simulink model "Core_Model_Controlled"  (R2023a)
settings: Solver=FixedStepAuto  StartTime=0.0  StopTime=Z  FixedStep=1/24  RelTol=1e-3
values from neighbouring files (symbols this model uses):
  c_eh = 0.85    [Model_Parameters.m]
  C_g = 1    [Model_Parameters.m]
  cc_e = -0.85    [Model_Parameters.m]
  id_a = 0.8*0.028*1.2    (= 0.02688)    [Model_Parameters.m]
  id_g = 0.8*0.072*1.2    (= 0.06912)    [Model_Parameters.m]
  id_l = 0.4*0.139*1.2    (= 0.06672)    [Model_Parameters.m]
  id_r = 0.4*0.428*1.2    (= 0.20544)    [Model_Parameters.m]
  id_z = 0.4*0.33*1.2    (= 0.1584)    [Model_Parameters.m]
  L_a = 0.25    [Model_Parameters.m]
  L_g = 0.1    [Model_Parameters.m]
  L_l = 0.2    [Model_Parameters.m]
  L_r = 0.05    [Model_Parameters.m]
  L_z = 0.08    [Model_Parameters.m]
  R_H2 = 0.05    [Model_Parameters.m]
  R_lh = 0.025    [Model_Parameters.m]
  R_ng = 0.025    [Model_Parameters.m]
  SF_MWh = SF_GWh*1e3    [Main_Script.m]
libraries: fl_lib x120, nesl_utility x93, ee_lib x36, slpidlib x1
(part 3 of 3)

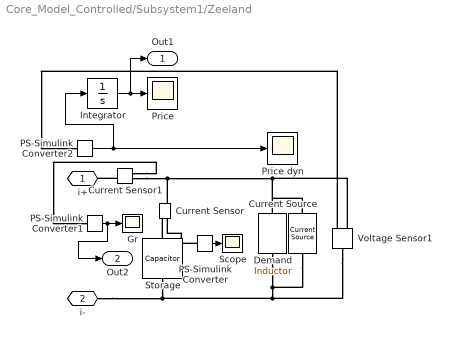
== system Core_Model_Controlled/Subsystem1/Zeeland ==
  Current Sensor : fl_lib/Electrical/Electrical Sensors/Current Sensor
  Current Sensor1 : fl_lib/Electrical/Electrical Sensors/Current Sensor
  Current Source : ee_lib/Sources/Current Source  dc_current=id_z A  ac_current=0 A  ac_shift=0 rad  ac_frequency=0 Hz  noise_mode=ee.enum.sources.noise.Disabled  PSD=0 A^2/Hz  sample_time=1e-3 s  repeatability=ee.enum.sources.repeatability.NotRepeatable  user_seed=0  auto_seed=4168664255  i_specify=off  i_priority=None  i=0 A  i_nominal_specify=off  i_nominal_unit=A  i_nominal_value=1  v_specify=off  v_priority=None  v=0 V  v_nominal_specify=off  v_nominal_unit=V  v_nominal_value=1
  Demand : ee_lib/Passive/Inductor  l=L_z H  enable_L_tol=0  L_tol=20  tol_distribution=1  nSigma=4  r=0 Ohm  g=0 1/Ohm  enable_operating_limits=0  operating_limit_action=2  max_working_current=1 A  power_rating=1 W  enable_faults=ee.enum.enable.no  fault_action=simscape.enum.assert.action.none  lambdaPercent=50  k_faulted=0.9999  turnsShort=0  openCct=0  groundShort=0  groundShortG=0 1/Ohm  tau_fault=1e-3 s  fault_trigger=ee.enum.faults.faultTrigger.temporal  t_fault=1 s  max_permissible_voltage=100 V  n_fail_on_voltage=1  max_permissible_current=1 A  t_fail_on_current=1 s  i_L_specify=off  i_L_priority=High  i_L=0 A  i_L_nominal_specify=off  i_L_nominal_unit=A  i_L_nominal_value=1
  Gr : Scope
  Integrator : Integrator
  PS-Simulink Converter : nesl_utility/PS-Simulink Converter  PhysicalDomain=network_engine_domain  SubClassName=ps_output  LeftPortType=input  RightPortType=output  PseudoPeriodic=off  Frequencies=[]  VectorFormat=inherit  Unit=inherit  AffineConversion=off
  PS-Simulink Converter1 : nesl_utility/PS-Simulink Converter  PhysicalDomain=network_engine_domain  SubClassName=ps_output  LeftPortType=input  RightPortType=output  PseudoPeriodic=off  Frequencies=[]  VectorFormat=inherit  Unit=inherit  AffineConversion=off
  PS-Simulink Converter2 : nesl_utility/PS-Simulink Converter  PhysicalDomain=network_engine_domain  SubClassName=ps_output  LeftPortType=input  RightPortType=output  PseudoPeriodic=off  Frequencies=[]  VectorFormat=inherit  Unit=inherit  AffineConversion=off
  "Price " : Scope
  Price dyn : Scope
  Scope : Scope
  Storage : fl_lib/Electrical/Electrical Elements/Capacitor  c=C_z F  r=0 Ohm  g=0 1/Ohm  i_specify=off  i_priority=None  i=0 A  i_nominal_specify=off  i_nominal_unit=A  i_nominal_value=1  v_specify=off  v_priority=None  v=0 V  v_nominal_specify=off  v_nominal_unit=V  v_nominal_value=1  vc_specify=off  vc_priority=High  vc=0 V  vc_nominal_specify=off  vc_nominal_unit=V  vc_nominal_value=1
  Voltage Sensor1 : fl_lib/Electrical/Electrical Sensors/Voltage Sensor
  "i+ " : PMIOPort  Tag=PMCPort  Side=Left
  i- : PMIOPort  Tag=PMCPort  Port=2  Side=Left
  Out1 : Outport
  Out2 : Outport  Port=2
  wires:
  Integrator/1 -> Out1/1, "Price "/1
  PS-Simulink Converter/1 -> Scope/1
  PS-Simulink Converter2/1 -> Integrator/1, Price dyn/1
  PS-Simulink Converter1/1 -> Out2/1, Gr/1
  connections:
  Demand/LConn1 -- Current Source/LConn1 -- i-/RConn1 -- Storage/LConn1 -- Voltage Sensor1/LConn1
  Current Sensor/LConn1 -- Voltage Sensor1/RConn2 -- Current Source/RConn1 -- Demand/RConn1 -- Current Sensor1/RConn2
  Storage/RConn1 -- Current Sensor/RConn2
  Voltage Sensor1/RConn1 -- PS-Simulink Converter2/LConn1
  PS-Simulink Converter/LConn1 -- Current Sensor/RConn1
  Current Sensor1/RConn1 -- PS-Simulink Converter1/LConn1
  Current Sensor1/LConn1 -- "i+ "/RConn1

== matlab function Core_Model_Controlled/Subsystem1/MATLAB Function1 ==
  data: X input; y output
function y = fcn(X)

% % y = 0.03*sin(0.3*X)*sign(sin(X))+0.03;
% 
T=3;

w=2*pi/T;
y = 0.3*sin(w*X);
y(y<0) = 0;


end




% T=3;
% 
% w=2*pi/T;
% y = cos(w*X);
% y(y<0) = 0;

== matlab function Core_Model_Controlled/Subsystem1/Yearly distribution1 ==
  data: wind_distr input; current output
function current= fcn(wind_distr)
wind=wind_distr;

%% Wind to Electricity

       
    % Power curve
    wind_speeds = [0, 2, 4, 6, 8, 10, 12, 14, 16, 18, 20, 22, 24, 26]; % Wind speed values
    power_output = [0, 0, 0.5, 1, 3.7, 4.7, 6.3, 9.5, 9.5, 9.5, 9.5, 9.5, 0, 0]; % Corresponding power output values  in MW
    %powercurve: https://www.researchgate.net/figure/Power-curve-of-the-Vestas-V164-95-turbine-including-some-technical-data-left-side-and_fig4_351600993

    % Interpolate the power curve
    power_curve = interp1(wind_speeds, power_output, wind, 'linear', 'extrap');  % 'extrap' for extrapolation MW/turbine = MW/9.5MW
    
    % Limit power output to positive values
    power_curve(power_curve < 0) = 0;

    % Apply the power curve to wind speed samples
    electricity_production = power_curve .* wind; %MW

    % Consider turbine availability and capacity if applicable
    availability_factor = 1; % Availability factor
    offshore_wind_capacity = 12e3; % Offshore wind capacity in MW (=10GW)
    nr_turbines=offshore_wind_capacity/9.5;
    % offshore_wind_capacity = 30; % Offshore wind capacity in MW

    % Produced electricity
    electricity_production_MW = electricity_production * availability_factor * nr_turbines; %MWh
    electricity_production_GW = electricity_production_MW*1e-3;

    %% Scaling to integrate within the model 
    % current = 2e7 * electricity_production;
    current = electricity_production_GW/26^2; %GWh/h

    % \ 0.0002*30/10*0.5
end

== matlab function Core_Model_Controlled/Subsystem/Yearly distribution1 ==
  data: wind_distr input; current output
function current= fcn(wind_distr)
wind=wind_distr;

%% Wind to Electricity

       
    % Power curve
    wind_speeds = [0, 2, 4, 6, 8, 10, 12, 14, 16, 18, 20, 22, 24, 26]; % Wind speed values
    power_output = [0, 0, 0.5, 1, 3.7, 4.7, 6.3, 9.5, 9.5, 9.5, 9.5, 9.5, 0, 0]; % Corresponding power output values  in MW
    %powercurve: https://www.researchgate.net/figure/Power-curve-of-the-Vestas-V164-95-turbine-including-some-technical-data-left-side-and_fig4_351600993

    % Interpolate the power curve
    power_curve = interp1(wind_speeds, power_output, wind, 'linear', 'extrap');  % 'extrap' for extrapolation MW/turbine = MW/9.5MW
    
    % Limit power output to positive values
    power_curve(power_curve < 0) = 0;

    % Apply the power curve to wind speed samples
    electricity_production = power_curve .* wind; %MW

    % Consider turbine availability and capacity if applicable
    availability_factor = 1; % Availability factor
    offshore_wind_capacity = 12e3; % Offshore wind capacity in MW (=10GW)
    nr_turbines=offshore_wind_capacity/9.5;
    % offshore_wind_capacity = 30; % Offshore wind capacity in MW

    % Produced electricity
    electricity_production_MW = electricity_production * availability_factor * nr_turbines; %MWh
    electricity_production_GW = electricity_production_MW*1e-3;

    %% Scaling to integrate within the model 
    % current = 2e7 * electricity_production;
    current = electricity_production_GW/26^2; %GWh/h

    % \ 0.0002*30/10*0.5
end

== matlab function Core_Model_Controlled/Subsystem1/NG Shock ==
  data: X input; y output
function y= fcn(X)

%% random steps
    if X >= 150 && X < 170
        y = -0.1;
    else
        y = 0;
    end

== matlab function Core_Model_Controlled/Subsystem1/LH2 Shock ==
  data: X input; y output
function y= fcn(X)

%% random steps
    if X >= 150 && X < 170
        y = -0.1;
    else
        y = 0;
    end

== matlab function Core_Model_Controlled/Subsystem/LH2 Shock1 ==
  data: X input; y output
function y= fcn(X)

%% random steps
    if X >= 150 && X < 170
        y = -0.1;
    else
        y = 0;
    end

== matlab function Core_Model_Controlled/Subsystem/MATLAB Function2 ==
  data: X input; y output
function y = fcn(X)

% % y = 0.03*sin(0.3*X)*sign(sin(X))+0.03;
% 
T=3;

w=2*pi/T;
y = 0.3*sin(w*X);
y(y<0) = 0;


end




% T=3;
% 
% w=2*pi/T;
% y = cos(w*X);
% y(y<0) = 0;

== matlab function Core_Model_Controlled/Subsystem/NG Shock1 ==
  data: X input; y output
function y= fcn(X)

%% random steps
    if X >= 150 && X < 170
        y = -0.1;
    else
        y = 0;
    end

== matlab function Core_Model_Controlled/Subsystem/Stochasticity (hourly)1 ==
  data: X input; hourly output
function hourly = fcn(X)

== matlab function Core_Model_Controlled/Subsystem/Wind Shock1 ==
  data: X input; y output
function y= fcn(X)

%% random steps
    if X >= 80 && X < 100
        y = 3;
    else
        y = 0;
    end

== matlab function Core_Model_Controlled/Subsystem/Yearly distribution2 ==
  data: X input; wind_distr output
function wind_distr= fcn(X)

%% Parameters
a0 = 9.564;
a1 = 1.636;
b1 = 0.4314;
a2 = 0.2612;
b2 = 0.2799;
a3 = -0.4869;
b3 = 0.4023;
a4 = -0.141;
b4 = 0.06985;
a5 = 0.1669;
b5 = 0.03972;
w = 0.01721;

% % c0 = 9.839;
% c1 = 0.2685;
% d1 = -0.1482;
% c2 = -0.08017;
% d2 = -0.08146;
% w2 = 6.288;


       aa0 =       10.21  ;
       aa1 =      0.1631 ;
       bb1 =     -0.2515 ;
       aa2 =    -0.05622  ;
       bb2 =    -0.08132  ;
       aa3 =    -0.01446  ;
       bb3 =     0.01009  ;
       ww =      6.545;
%% Generate wind distributions
yearly_w = a0 + a1*cos(X*w) + b1*sin(X*w) + a2*cos(2*X*w) + b2*sin(2*X*w) + a3*cos(3*X*w) + b3*sin(3*X*w) + a4*cos(4*X*w) + b4*sin(4*X*w) + a5*cos(5*X*w) + b5*sin(5*X*w);
% daily_w = c1*cos(X*w2) + d1*sin(X*w2) + c2*cos(2*X*w2) + d2*sin(2*X*w2);


% Convert X from days to hours by dividing by 24
X_in_hours = X ;

daily_w =  aa1*cos(X_in_hours*ww) + bb1*sin(X_in_hours*ww) + aa2*cos(2*X_in_hours*ww) + bb2*sin(2*X_in_hours*ww) + aa3*cos(3*X_in_hours*ww) + bb3*sin(3*X_in_hours*ww);
    

% Total wind distribution
wind_distr = yearly_w + daily_w; %TNO: Offshore wind energy deployment in the North Sea by 2030: long-term measurement campaign.EPL, 2016-2020

end

== matlab function Core_Model_Controlled/Subsystem/Yearly distribution3 ==
  data: wind_distr input; current output; hourly input; step input
function current= fcn(wind_distr, hourly,step)
wind=wind_distr+hourly-step;

%% Wind to Electricity

       
    % Power curve
    wind_speeds = [0, 2, 4, 6, 8, 10, 12, 14, 16, 18, 20, 22, 24, 26]; % Wind speed values
    power_output = [0, 0, 0.5, 1, 3.7, 4.7, 6.3, 9.5, 9.5, 9.5, 9.5, 9.5, 0, 0]; % Corresponding power output values  in MW
    %powercurve: https://www.researchgate.net/figure/Power-curve-of-the-Vestas-V164-95-turbine-including-some-technical-data-left-side-and_fig4_351600993

    % Interpolate the power curve
    power_curve = interp1(wind_speeds, power_output, wind, 'linear', 'extrap');  % 'extrap' for extrapolation MW/turbine = MW/9.5MW
    
    % Limit power output to positive values
    power_curve(power_curve < 0) = 0;

    % Apply the power curve to wind speed samples
    electricity_production = power_curve .* wind; %MW

    % Consider turbine availability and capacity if applicable
    availability_factor = 1; % Availability factor
    offshore_wind_capacity = 12e3; % Offshore wind capacity in MW (=10GW)
    nr_turbines=offshore_wind_capacity/9.5;
    % offshore_wind_capacity = 30; % Offshore wind capacity in MW

    % Produced electricity
    electricity_production_MW = electricity_production * availability_factor * nr_turbines; %MWh
    electricity_production_GW = electricity_production_MW*1e-3;

    %% Scaling to integrate within the model 
    % current = 2e7 * electricity_production;
    current = electricity_production_GW/26^2; %GWh/h

    % \ 0.0002*30/10*0.5
end
